simulink model "PIRegler_Spin"  (R2022a)
settings: Solver=VariableStepAuto  StartTime=0.0  StopTime=10.0  RelTol=1e-3
libraries: cstblocks x1
settings Model: Creator=Uni  LastModifiedBy=Uni

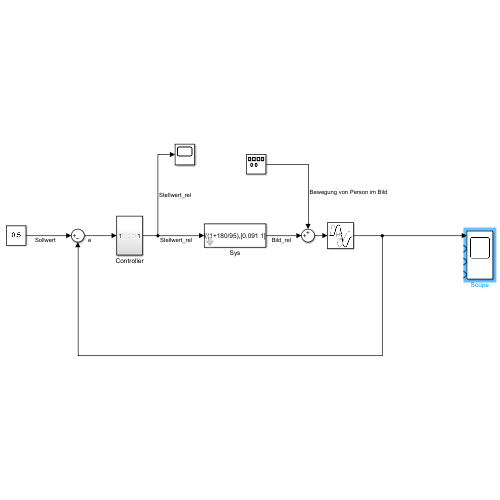
[thumbnail: Simulink's stored preview of the top-level diagram]
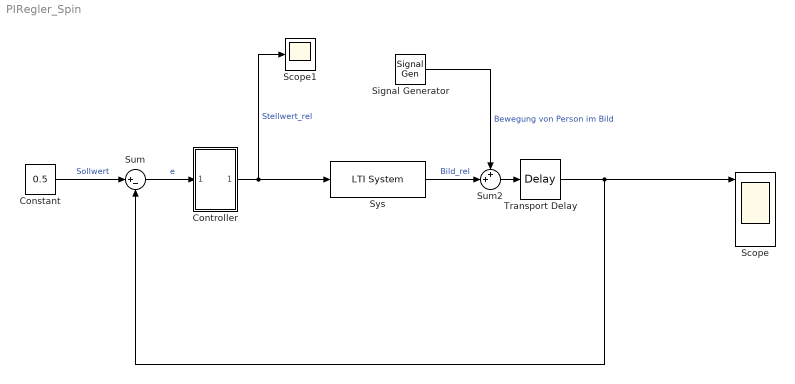
== system PIRegler_Spin ==
  Constant : Constant  Value=0.5
  Controller : Subsystem
  Scope : Scope  NumInputPorts=4
  Scope1 : Scope
  Signal Generator : SignalGenerator  Amplitude=0.5  Units=rad/sec
  Sum : Sum  Inputs=|+-
  Sum2 : Sum  Inputs=++|
  Sys : cstblocks/LTI System  sys=tf((1+180/95),[0.091 1])  IC=[]
  Transport Delay : TransportDelay  DelayTime=0.65
  wires:
  Signal Generator/1 -> Sum2/1  "Bewegung von Person im Bild"
  Transport Delay/1 -> Sum/2, Scope/1
  Sys/1 -> Sum2/2  "Bild_rel"
  Sum/1 -> Controller/1(In2)  "e"
  Controller/1(Out2) -> Sys/1, Scope1/1  "Stellwert_rel"
  Constant/1 -> Sum/1  "Sollwert"
  Sum2/1 -> Transport Delay/1

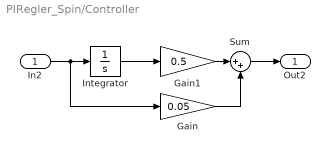
== system PIRegler_Spin/Controller ==
  In2 : Inport
  Gain : Gain  Gain=0.05
  Gain1 : Gain  Gain=0.5
  Integrator : Integrator
  Sum : Sum  Inputs=|++
  Out2 : Outport
  wires:
  Gain1/1 -> Sum/1
  Gain/1 -> Sum/2
  Integrator/1 -> Gain1/1
  In2/1 -> Integrator/1, Gain/1
  Sum/1 -> Out2/1
